simulink model "tx2"  (R2022a)
settings: Solver=FixedStepDiscrete  StartTime=0.0  StopTime=3.1e6  FixedStep=1  RelTol=1e-3
undefined symbols (not defined in the file or in its folder): rom_bf1, rom_bf2, rom_bf3, rom_bf4, rom_bf5, rom_bf6, rom_bf7, rom_bf8, rom_pilot_tt
libraries: hdlsllib x809, whdlutilities x460, whdlmod x104, whdledac x26, simulink x3
(part 2 of 27)

== system tx2/Subsystem1 ==
  process_data : Inport
  process_valid : Inport  Port=2
  BF : Subsystem
      settings: PortSchema="{\"entries\":[{\"content\":{\"sides\":[{\"content\":{\"connectorIds\":[\"In1\",\"In2\"]},\"type\":\"ConnectorPlacement.EquallySpacedRectSide\",\"uuid\":\"594cb7fb-008e-4551-8b9f-b11ed50deaba\"},{\"content\":{\"connectorIds\":[\"Out1\",\"Out2\",\"Out3\"],\"side\":\"RIGHT\"},\"type\":\"ConnectorPlacement.EquallySpacedRectSide\",\"uuid\":\"93ae86ad-1f5c-4115-9520-3a1a0cabfd8c\"},{\"content\":{\"connectorIds\":[\"In3\",\"In4\"],\"side\":\"TOP\"},\"type\":\"ConnectorPlacement.EquallySpacedRectSide\",\"uuid\":\"1fce8a66-8094-4bbb-b964-246637a8c1f4\"},{\"content\":{\"connectorIds\":[],\"side\":\"BOTTOM\"},\"type\":\"ConnectorPlacement.EquallySpacedRectSide\",\"uuid\":\"d45d1c11-e328-4038-90b1-bd9740dff9db\"}]},\"type\":\"ConnectorPlacement.EquallySpacedConnector\",\"uuid\":\"0bd8d214-ca11-4ecb-a7f0-3e13fd4fb1b3\"}],\"packageUris\":[\"http://schema.mathworks.com/mf0/Connector/R2020b\"],\"version\":\"1.0\"}"
  Bus Creator : BusCreator  Inputs=8
  Mux : Mux  Inputs=8
  OFDM_process1 : Subsystem  mask{cp=72}
      mask prompts: cp "the length of cp"
      mask DialogControl ParameterGroupVar Prompt: 参数
  bit_level : Subsystem
  mapping_process_L1 : Subsystem
      settings: PortSchema="{\"entries\":[{\"content\":{\"sides\":[{\"content\":{\"connectorIds\":[\"In1\",\"In2\"]},\"type\":\"ConnectorPlacement.EquallySpacedRectSide\",\"uuid\":\"660ebed9-a9a7-400e-a1e1-2a3bed22b258\"},{\"content\":{\"connectorIds\":[\"Out1\",\"Out2\"],\"side\":\"RIGHT\"},\"type\":\"ConnectorPlacement.EquallySpacedRectSide\",\"uuid\":\"141e197b-598d-477b-8a8c-cee3f2454319\"},{\"content\":{\"connectorIds\":[\"Out3\",\"Out4\"],\"side\":\"TOP\"},\"type\":\"ConnectorPlacement.EquallySpacedRectSide\",\"uuid\":\"c80a2ec3-9c02-4c14-8d74-14079e138b72\"}]},\"type\":\"ConnectorPlacement.EquallySpacedConnector\",\"uuid\":\"42120fb8-a7c5-4b68-b1ff-3dfc935ed9da\"}],\"packageUris\":[\"http://schema.mathworks.com/mf0/Connector/R2020b\"],\"version\":\"1.0\"}"
  OFDM_bf : Outport  PortDimensions=8
  OFDM_ctrl_bf : Outport  Port=2  OutDataTypeStr=Bus: BUSOFDM2
  wires:
  bit_level/2("bit_level_ctrl_process ") -> mapping_process_L1/2(mapping_ctrl)  "bit_level_ctrl"
  process_data/1 -> bit_level/1(process_data)
  mapping_process_L1/4(RB_id) -> BF/3(RB_id)  "RB_id_L1"
  mapping_process_L1/2(ctrl_mapping) -> BF/2(BF_data_ctrl)  "ctrl_mapping"
  mapping_process_L1/3(RB_ctrl) -> BF/4(RB_id_ctrl)  "RB_ctrl"
  bit_level/1(bit_level_process) -> mapping_process_L1/1(data_in)  "bit_level_process1"
  mapping_process_L1/1(data_out) -> BF/1(layer_data_in1)  "mapping_data_L1"
  process_valid/1 -> bit_level/2(process_valid)
  OFDM_process1/15(OFDM_bf8) -> Mux/8
  OFDM_process1/8(OFDM_ctrl_bf4) -> Bus Creator/4  "L4"
  OFDM_process1/1(OFDM_bf1) -> Mux/1
  OFDM_process1/5(OFDM_bf3) -> Mux/3
  Bus Creator/1 -> OFDM_ctrl_bf/1
  Mux/1 -> OFDM_bf/1
  BF/2(BF_ctrl) -> OFDM_process1/2(BF_ctrl)  "BF_ctrl"
  OFDM_process1/16(OFDM_ctrl_bf8) -> Bus Creator/8  "L8"
  OFDM_process1/10(OFDM_ctrl_bf5) -> Bus Creator/5  "L5"
  OFDM_process1/14(OFDM_ctrl_bf7) -> Bus Creator/7  "L7"
  OFDM_process1/12(OFDM_ctrl_bf6) -> Bus Creator/6  "L6"
  OFDM_process1/11(OFDM_bf6) -> Mux/6
  OFDM_process1/13(OFDM_bf7) -> Mux/7
  OFDM_process1/4(OFDM_ctrl_bf2) -> Bus Creator/2  "L2"
  OFDM_process1/3(OFDM_bf2) -> Mux/2
  OFDM_process1/7(OFDM_bf4) -> Mux/4
  OFDM_process1/9(OFDM_bf5) -> Mux/5
  OFDM_process1/2(OFDM_ctrl_bf1) -> Bus Creator/1  "L1"
  OFDM_process1/6(OFDM_ctrl_bf3) -> Bus Creator/3  "L3"
  BF/1(process_bf) -> OFDM_process1/1(process_bf)  "process_bf"

== system tx2/Subsystem10 ==
  process_data : Inport
  process_valid : Inport  Port=2
  BF : Subsystem
      settings: PortSchema="{\"entries\":[{\"content\":{\"sides\":[{\"content\":{\"connectorIds\":[\"In1\",\"In2\"]},\"type\":\"ConnectorPlacement.EquallySpacedRectSide\",\"uuid\":\"594cb7fb-008e-4551-8b9f-b11ed50deaba\"},{\"content\":{\"connectorIds\":[\"Out1\",\"Out2\",\"Out3\"],\"side\":\"RIGHT\"},\"type\":\"ConnectorPlacement.EquallySpacedRectSide\",\"uuid\":\"93ae86ad-1f5c-4115-9520-3a1a0cabfd8c\"},{\"content\":{\"connectorIds\":[\"In3\",\"In4\"],\"side\":\"TOP\"},\"type\":\"ConnectorPlacement.EquallySpacedRectSide\",\"uuid\":\"1fce8a66-8094-4bbb-b964-246637a8c1f4\"},{\"content\":{\"connectorIds\":[],\"side\":\"BOTTOM\"},\"type\":\"ConnectorPlacement.EquallySpacedRectSide\",\"uuid\":\"d45d1c11-e328-4038-90b1-bd9740dff9db\"}]},\"type\":\"ConnectorPlacement.EquallySpacedConnector\",\"uuid\":\"0bd8d214-ca11-4ecb-a7f0-3e13fd4fb1b3\"}],\"packageUris\":[\"http://schema.mathworks.com/mf0/Connector/R2020b\"],\"version\":\"1.0\"}"
  Bus Creator : BusCreator  Inputs=8
  Mux : Mux  Inputs=8
  OFDM_process1 : Subsystem  mask{cp=72}
      mask prompts: cp "the length of cp"
      mask DialogControl ParameterGroupVar Prompt: 参数
  bit_level : Subsystem
  mapping_process_L1 : Subsystem
      settings: PortSchema="{\"entries\":[{\"content\":{\"sides\":[{\"content\":{\"connectorIds\":[\"In1\",\"In2\"]},\"type\":\"ConnectorPlacement.EquallySpacedRectSide\",\"uuid\":\"660ebed9-a9a7-400e-a1e1-2a3bed22b258\"},{\"content\":{\"connectorIds\":[\"Out1\",\"Out2\"],\"side\":\"RIGHT\"},\"type\":\"ConnectorPlacement.EquallySpacedRectSide\",\"uuid\":\"141e197b-598d-477b-8a8c-cee3f2454319\"},{\"content\":{\"connectorIds\":[\"Out3\",\"Out4\"],\"side\":\"TOP\"},\"type\":\"ConnectorPlacement.EquallySpacedRectSide\",\"uuid\":\"c80a2ec3-9c02-4c14-8d74-14079e138b72\"}]},\"type\":\"ConnectorPlacement.EquallySpacedConnector\",\"uuid\":\"42120fb8-a7c5-4b68-b1ff-3dfc935ed9da\"}],\"packageUris\":[\"http://schema.mathworks.com/mf0/Connector/R2020b\"],\"version\":\"1.0\"}"
  OFDM_bf : Outport  PortDimensions=8
  OFDM_ctrl_bf : Outport  Port=2  OutDataTypeStr=Bus: BUSOFDM2
  wires:
  BF/1(process_bf) -> OFDM_process1/1(process_bf)  "process_bf"
  OFDM_process1/6(OFDM_ctrl_bf3) -> Bus Creator/3  "L3"
  OFDM_process1/2(OFDM_ctrl_bf1) -> Bus Creator/1  "L1"
  OFDM_process1/9(OFDM_bf5) -> Mux/5
  OFDM_process1/7(OFDM_bf4) -> Mux/4
  OFDM_process1/3(OFDM_bf2) -> Mux/2
  OFDM_process1/4(OFDM_ctrl_bf2) -> Bus Creator/2  "L2"
  OFDM_process1/13(OFDM_bf7) -> Mux/7
  OFDM_process1/11(OFDM_bf6) -> Mux/6
  OFDM_process1/12(OFDM_ctrl_bf6) -> Bus Creator/6  "L6"
  OFDM_process1/14(OFDM_ctrl_bf7) -> Bus Creator/7  "L7"
  OFDM_process1/10(OFDM_ctrl_bf5) -> Bus Creator/5  "L5"
  OFDM_process1/16(OFDM_ctrl_bf8) -> Bus Creator/8  "L8"
  BF/2(BF_ctrl) -> OFDM_process1/2(BF_ctrl)  "BF_ctrl"
  Mux/1 -> OFDM_bf/1
  Bus Creator/1 -> OFDM_ctrl_bf/1
  OFDM_process1/5(OFDM_bf3) -> Mux/3
  OFDM_process1/1(OFDM_bf1) -> Mux/1
  OFDM_process1/8(OFDM_ctrl_bf4) -> Bus Creator/4  "L4"
  OFDM_process1/15(OFDM_bf8) -> Mux/8
  process_valid/1 -> bit_level/2(process_valid)
  mapping_process_L1/1(data_out) -> BF/1(layer_data_in1)  "mapping_data_L1"
  bit_level/1(bit_level_process) -> mapping_process_L1/1(data_in)  "bit_level_process1"
  mapping_process_L1/3(RB_ctrl) -> BF/4(RB_id_ctrl)  "RB_ctrl"
  mapping_process_L1/2(ctrl_mapping) -> BF/2(BF_data_ctrl)  "ctrl_mapping"
  mapping_process_L1/4(RB_id) -> BF/3(RB_id)  "RB_id_L1"
  process_data/1 -> bit_level/1(process_data)
  bit_level/2("bit_level_ctrl_process ") -> mapping_process_L1/2(mapping_ctrl)  "bit_level_ctrl"

== system tx2/Subsystem11 ==
  process_data : Inport
  process_valid : Inport  Port=2
  BF : Subsystem
      settings: PortSchema="{\"entries\":[{\"content\":{\"sides\":[{\"content\":{\"connectorIds\":[\"In1\",\"In2\"]},\"type\":\"ConnectorPlacement.EquallySpacedRectSide\",\"uuid\":\"594cb7fb-008e-4551-8b9f-b11ed50deaba\"},{\"content\":{\"connectorIds\":[\"Out1\",\"Out2\",\"Out3\"],\"side\":\"RIGHT\"},\"type\":\"ConnectorPlacement.EquallySpacedRectSide\",\"uuid\":\"93ae86ad-1f5c-4115-9520-3a1a0cabfd8c\"},{\"content\":{\"connectorIds\":[\"In3\",\"In4\"],\"side\":\"TOP\"},\"type\":\"ConnectorPlacement.EquallySpacedRectSide\",\"uuid\":\"1fce8a66-8094-4bbb-b964-246637a8c1f4\"},{\"content\":{\"connectorIds\":[],\"side\":\"BOTTOM\"},\"type\":\"ConnectorPlacement.EquallySpacedRectSide\",\"uuid\":\"d45d1c11-e328-4038-90b1-bd9740dff9db\"}]},\"type\":\"ConnectorPlacement.EquallySpacedConnector\",\"uuid\":\"0bd8d214-ca11-4ecb-a7f0-3e13fd4fb1b3\"}],\"packageUris\":[\"http://schema.mathworks.com/mf0/Connector/R2020b\"],\"version\":\"1.0\"}"
  Bus Creator : BusCreator  Inputs=8
  Mux : Mux  Inputs=8
  OFDM_process1 : Subsystem  mask{cp=72}
      mask prompts: cp "the length of cp"
      mask DialogControl ParameterGroupVar Prompt: 参数
  bit_level : Subsystem
  mapping_process_L1 : Subsystem
      settings: PortSchema="{\"entries\":[{\"content\":{\"sides\":[{\"content\":{\"connectorIds\":[\"In1\",\"In2\"]},\"type\":\"ConnectorPlacement.EquallySpacedRectSide\",\"uuid\":\"660ebed9-a9a7-400e-a1e1-2a3bed22b258\"},{\"content\":{\"connectorIds\":[\"Out1\",\"Out2\"],\"side\":\"RIGHT\"},\"type\":\"ConnectorPlacement.EquallySpacedRectSide\",\"uuid\":\"141e197b-598d-477b-8a8c-cee3f2454319\"},{\"content\":{\"connectorIds\":[\"Out3\",\"Out4\"],\"side\":\"TOP\"},\"type\":\"ConnectorPlacement.EquallySpacedRectSide\",\"uuid\":\"c80a2ec3-9c02-4c14-8d74-14079e138b72\"}]},\"type\":\"ConnectorPlacement.EquallySpacedConnector\",\"uuid\":\"42120fb8-a7c5-4b68-b1ff-3dfc935ed9da\"}],\"packageUris\":[\"http://schema.mathworks.com/mf0/Connector/R2020b\"],\"version\":\"1.0\"}"
  OFDM_bf : Outport  PortDimensions=8
  OFDM_ctrl_bf : Outport  Port=2  OutDataTypeStr=Bus: BUSOFDM2
  wires:
  bit_level/2("bit_level_ctrl_process ") -> mapping_process_L1/2(mapping_ctrl)  "bit_level_ctrl"
  process_data/1 -> bit_level/1(process_data)
  mapping_process_L1/4(RB_id) -> BF/3(RB_id)  "RB_id_L1"
  mapping_process_L1/2(ctrl_mapping) -> BF/2(BF_data_ctrl)  "ctrl_mapping"
  mapping_process_L1/3(RB_ctrl) -> BF/4(RB_id_ctrl)  "RB_ctrl"
  bit_level/1(bit_level_process) -> mapping_process_L1/1(data_in)  "bit_level_process1"
  mapping_process_L1/1(data_out) -> BF/1(layer_data_in1)  "mapping_data_L1"
  process_valid/1 -> bit_level/2(process_valid)
  OFDM_process1/15(OFDM_bf8) -> Mux/8
  OFDM_process1/8(OFDM_ctrl_bf4) -> Bus Creator/4  "L4"
  OFDM_process1/1(OFDM_bf1) -> Mux/1
  OFDM_process1/5(OFDM_bf3) -> Mux/3
  Bus Creator/1 -> OFDM_ctrl_bf/1
  Mux/1 -> OFDM_bf/1
  BF/2(BF_ctrl) -> OFDM_process1/2(BF_ctrl)  "BF_ctrl"
  OFDM_process1/16(OFDM_ctrl_bf8) -> Bus Creator/8  "L8"
  OFDM_process1/10(OFDM_ctrl_bf5) -> Bus Creator/5  "L5"
  OFDM_process1/14(OFDM_ctrl_bf7) -> Bus Creator/7  "L7"
  OFDM_process1/12(OFDM_ctrl_bf6) -> Bus Creator/6  "L6"
  OFDM_process1/11(OFDM_bf6) -> Mux/6
  OFDM_process1/13(OFDM_bf7) -> Mux/7
  OFDM_process1/4(OFDM_ctrl_bf2) -> Bus Creator/2  "L2"
  OFDM_process1/3(OFDM_bf2) -> Mux/2
  OFDM_process1/7(OFDM_bf4) -> Mux/4
  OFDM_process1/9(OFDM_bf5) -> Mux/5
  OFDM_process1/2(OFDM_ctrl_bf1) -> Bus Creator/1  "L1"
  OFDM_process1/6(OFDM_ctrl_bf3) -> Bus Creator/3  "L3"
  BF/1(process_bf) -> OFDM_process1/1(process_bf)  "process_bf"

== system tx2/Subsystem12 ==
  process_data : Inport
  process_valid : Inport  Port=2
  BF : Subsystem
      settings: PortSchema="{\"entries\":[{\"content\":{\"sides\":[{\"content\":{\"connectorIds\":[\"In1\",\"In2\"]},\"type\":\"ConnectorPlacement.EquallySpacedRectSide\",\"uuid\":\"594cb7fb-008e-4551-8b9f-b11ed50deaba\"},{\"content\":{\"connectorIds\":[\"Out1\",\"Out2\",\"Out3\"],\"side\":\"RIGHT\"},\"type\":\"ConnectorPlacement.EquallySpacedRectSide\",\"uuid\":\"93ae86ad-1f5c-4115-9520-3a1a0cabfd8c\"},{\"content\":{\"connectorIds\":[\"In3\",\"In4\"],\"side\":\"TOP\"},\"type\":\"ConnectorPlacement.EquallySpacedRectSide\",\"uuid\":\"1fce8a66-8094-4bbb-b964-246637a8c1f4\"},{\"content\":{\"connectorIds\":[],\"side\":\"BOTTOM\"},\"type\":\"ConnectorPlacement.EquallySpacedRectSide\",\"uuid\":\"d45d1c11-e328-4038-90b1-bd9740dff9db\"}]},\"type\":\"ConnectorPlacement.EquallySpacedConnector\",\"uuid\":\"0bd8d214-ca11-4ecb-a7f0-3e13fd4fb1b3\"}],\"packageUris\":[\"http://schema.mathworks.com/mf0/Connector/R2020b\"],\"version\":\"1.0\"}"
  Bus Creator : BusCreator  Inputs=8
  Mux : Mux  Inputs=8
  OFDM_process1 : Subsystem  mask{cp=72}
      mask prompts: cp "the length of cp"
      mask DialogControl ParameterGroupVar Prompt: 参数
  bit_level : Subsystem
  mapping_process_L1 : Subsystem
      settings: PortSchema="{\"entries\":[{\"content\":{\"sides\":[{\"content\":{\"connectorIds\":[\"In1\",\"In2\"]},\"type\":\"ConnectorPlacement.EquallySpacedRectSide\",\"uuid\":\"660ebed9-a9a7-400e-a1e1-2a3bed22b258\"},{\"content\":{\"connectorIds\":[\"Out1\",\"Out2\"],\"side\":\"RIGHT\"},\"type\":\"ConnectorPlacement.EquallySpacedRectSide\",\"uuid\":\"141e197b-598d-477b-8a8c-cee3f2454319\"},{\"content\":{\"connectorIds\":[\"Out3\",\"Out4\"],\"side\":\"TOP\"},\"type\":\"ConnectorPlacement.EquallySpacedRectSide\",\"uuid\":\"c80a2ec3-9c02-4c14-8d74-14079e138b72\"}]},\"type\":\"ConnectorPlacement.EquallySpacedConnector\",\"uuid\":\"42120fb8-a7c5-4b68-b1ff-3dfc935ed9da\"}],\"packageUris\":[\"http://schema.mathworks.com/mf0/Connector/R2020b\"],\"version\":\"1.0\"}"
  OFDM_bf : Outport  PortDimensions=8
  OFDM_ctrl_bf : Outport  Port=2  OutDataTypeStr=Bus: BUSOFDM2
  wires:
  BF/1(process_bf) -> OFDM_process1/1(process_bf)  "process_bf"
  OFDM_process1/6(OFDM_ctrl_bf3) -> Bus Creator/3  "L3"
  OFDM_process1/2(OFDM_ctrl_bf1) -> Bus Creator/1  "L1"
  OFDM_process1/9(OFDM_bf5) -> Mux/5
  OFDM_process1/7(OFDM_bf4) -> Mux/4
  OFDM_process1/3(OFDM_bf2) -> Mux/2
  OFDM_process1/4(OFDM_ctrl_bf2) -> Bus Creator/2  "L2"
  OFDM_process1/13(OFDM_bf7) -> Mux/7
  OFDM_process1/11(OFDM_bf6) -> Mux/6
  OFDM_process1/12(OFDM_ctrl_bf6) -> Bus Creator/6  "L6"
  OFDM_process1/14(OFDM_ctrl_bf7) -> Bus Creator/7  "L7"
  OFDM_process1/10(OFDM_ctrl_bf5) -> Bus Creator/5  "L5"
  OFDM_process1/16(OFDM_ctrl_bf8) -> Bus Creator/8  "L8"
  BF/2(BF_ctrl) -> OFDM_process1/2(BF_ctrl)  "BF_ctrl"
  Mux/1 -> OFDM_bf/1
  Bus Creator/1 -> OFDM_ctrl_bf/1
  OFDM_process1/5(OFDM_bf3) -> Mux/3
  OFDM_process1/1(OFDM_bf1) -> Mux/1
  OFDM_process1/8(OFDM_ctrl_bf4) -> Bus Creator/4  "L4"
  OFDM_process1/15(OFDM_bf8) -> Mux/8
  process_valid/1 -> bit_level/2(process_valid)
  mapping_process_L1/1(data_out) -> BF/1(layer_data_in1)  "mapping_data_L1"
  bit_level/1(bit_level_process) -> mapping_process_L1/1(data_in)  "bit_level_process1"
  mapping_process_L1/3(RB_ctrl) -> BF/4(RB_id_ctrl)  "RB_ctrl"
  mapping_process_L1/2(ctrl_mapping) -> BF/2(BF_data_ctrl)  "ctrl_mapping"
  mapping_process_L1/4(RB_id) -> BF/3(RB_id)  "RB_id_L1"
  process_data/1 -> bit_level/1(process_data)
  bit_level/2("bit_level_ctrl_process ") -> mapping_process_L1/2(mapping_ctrl)  "bit_level_ctrl"

== system tx2/Subsystem13 ==
  process_data : Inport
  process_valid : Inport  Port=2
  BF : Subsystem
      settings: PortSchema="{\"entries\":[{\"content\":{\"sides\":[{\"content\":{\"connectorIds\":[\"In1\",\"In2\"]},\"type\":\"ConnectorPlacement.EquallySpacedRectSide\",\"uuid\":\"594cb7fb-008e-4551-8b9f-b11ed50deaba\"},{\"content\":{\"connectorIds\":[\"Out1\",\"Out2\",\"Out3\"],\"side\":\"RIGHT\"},\"type\":\"ConnectorPlacement.EquallySpacedRectSide\",\"uuid\":\"93ae86ad-1f5c-4115-9520-3a1a0cabfd8c\"},{\"content\":{\"connectorIds\":[\"In3\",\"In4\"],\"side\":\"TOP\"},\"type\":\"ConnectorPlacement.EquallySpacedRectSide\",\"uuid\":\"1fce8a66-8094-4bbb-b964-246637a8c1f4\"},{\"content\":{\"connectorIds\":[],\"side\":\"BOTTOM\"},\"type\":\"ConnectorPlacement.EquallySpacedRectSide\",\"uuid\":\"d45d1c11-e328-4038-90b1-bd9740dff9db\"}]},\"type\":\"ConnectorPlacement.EquallySpacedConnector\",\"uuid\":\"0bd8d214-ca11-4ecb-a7f0-3e13fd4fb1b3\"}],\"packageUris\":[\"http://schema.mathworks.com/mf0/Connector/R2020b\"],\"version\":\"1.0\"}"
  Bus Creator : BusCreator  Inputs=8
  Mux : Mux  Inputs=8
  OFDM_process1 : Subsystem  mask{cp=72}
      mask prompts: cp "the length of cp"
      mask DialogControl ParameterGroupVar Prompt: 参数
  bit_level : Subsystem
  mapping_process_L1 : Subsystem
      settings: PortSchema="{\"entries\":[{\"content\":{\"sides\":[{\"content\":{\"connectorIds\":[\"In1\",\"In2\"]},\"type\":\"ConnectorPlacement.EquallySpacedRectSide\",\"uuid\":\"660ebed9-a9a7-400e-a1e1-2a3bed22b258\"},{\"content\":{\"connectorIds\":[\"Out1\",\"Out2\"],\"side\":\"RIGHT\"},\"type\":\"ConnectorPlacement.EquallySpacedRectSide\",\"uuid\":\"141e197b-598d-477b-8a8c-cee3f2454319\"},{\"content\":{\"connectorIds\":[\"Out3\",\"Out4\"],\"side\":\"TOP\"},\"type\":\"ConnectorPlacement.EquallySpacedRectSide\",\"uuid\":\"c80a2ec3-9c02-4c14-8d74-14079e138b72\"}]},\"type\":\"ConnectorPlacement.EquallySpacedConnector\",\"uuid\":\"42120fb8-a7c5-4b68-b1ff-3dfc935ed9da\"}],\"packageUris\":[\"http://schema.mathworks.com/mf0/Connector/R2020b\"],\"version\":\"1.0\"}"
  OFDM_bf : Outport  PortDimensions=8
  OFDM_ctrl_bf : Outport  Port=2  OutDataTypeStr=Bus: BUSOFDM2
  wires:
  bit_level/2("bit_level_ctrl_process ") -> mapping_process_L1/2(mapping_ctrl)  "bit_level_ctrl"
  process_data/1 -> bit_level/1(process_data)
  mapping_process_L1/4(RB_id) -> BF/3(RB_id)  "RB_id_L1"
  mapping_process_L1/2(ctrl_mapping) -> BF/2(BF_data_ctrl)  "ctrl_mapping"
  mapping_process_L1/3(RB_ctrl) -> BF/4(RB_id_ctrl)  "RB_ctrl"
  bit_level/1(bit_level_process) -> mapping_process_L1/1(data_in)  "bit_level_process1"
  mapping_process_L1/1(data_out) -> BF/1(layer_data_in1)  "mapping_data_L1"
  process_valid/1 -> bit_level/2(process_valid)
  OFDM_process1/15(OFDM_bf8) -> Mux/8
  OFDM_process1/8(OFDM_ctrl_bf4) -> Bus Creator/4  "L4"
  OFDM_process1/1(OFDM_bf1) -> Mux/1
  OFDM_process1/5(OFDM_bf3) -> Mux/3
  Bus Creator/1 -> OFDM_ctrl_bf/1
  Mux/1 -> OFDM_bf/1
  BF/2(BF_ctrl) -> OFDM_process1/2(BF_ctrl)  "BF_ctrl"
  OFDM_process1/16(OFDM_ctrl_bf8) -> Bus Creator/8  "L8"
  OFDM_process1/10(OFDM_ctrl_bf5) -> Bus Creator/5  "L5"
  OFDM_process1/14(OFDM_ctrl_bf7) -> Bus Creator/7  "L7"
  OFDM_process1/12(OFDM_ctrl_bf6) -> Bus Creator/6  "L6"
  OFDM_process1/11(OFDM_bf6) -> Mux/6
  OFDM_process1/13(OFDM_bf7) -> Mux/7
  OFDM_process1/4(OFDM_ctrl_bf2) -> Bus Creator/2  "L2"
  OFDM_process1/3(OFDM_bf2) -> Mux/2
  OFDM_process1/7(OFDM_bf4) -> Mux/4
  OFDM_process1/9(OFDM_bf5) -> Mux/5
  OFDM_process1/2(OFDM_ctrl_bf1) -> Bus Creator/1  "L1"
  OFDM_process1/6(OFDM_ctrl_bf3) -> Bus Creator/3  "L3"
  BF/1(process_bf) -> OFDM_process1/1(process_bf)  "process_bf"

== system tx2/Subsystem2 ==
  process_data : Inport
  process_valid : Inport  Port=2
  BF : Subsystem
      settings: PortSchema="{\"entries\":[{\"content\":{\"sides\":[{\"content\":{\"connectorIds\":[\"In1\",\"In2\"]},\"type\":\"ConnectorPlacement.EquallySpacedRectSide\",\"uuid\":\"594cb7fb-008e-4551-8b9f-b11ed50deaba\"},{\"content\":{\"connectorIds\":[\"Out1\",\"Out2\",\"Out3\"],\"side\":\"RIGHT\"},\"type\":\"ConnectorPlacement.EquallySpacedRectSide\",\"uuid\":\"93ae86ad-1f5c-4115-9520-3a1a0cabfd8c\"},{\"content\":{\"connectorIds\":[\"In3\",\"In4\"],\"side\":\"TOP\"},\"type\":\"ConnectorPlacement.EquallySpacedRectSide\",\"uuid\":\"1fce8a66-8094-4bbb-b964-246637a8c1f4\"},{\"content\":{\"connectorIds\":[],\"side\":\"BOTTOM\"},\"type\":\"ConnectorPlacement.EquallySpacedRectSide\",\"uuid\":\"d45d1c11-e328-4038-90b1-bd9740dff9db\"}]},\"type\":\"ConnectorPlacement.EquallySpacedConnector\",\"uuid\":\"0bd8d214-ca11-4ecb-a7f0-3e13fd4fb1b3\"}],\"packageUris\":[\"http://schema.mathworks.com/mf0/Connector/R2020b\"],\"version\":\"1.0\"}"
  Bus Creator : BusCreator  Inputs=8
  Mux : Mux  Inputs=8
  OFDM_process1 : Subsystem  mask{cp=72}
      mask prompts: cp "the length of cp"
      mask DialogControl ParameterGroupVar Prompt: 参数
  bit_level : Subsystem
  mapping_process_L1 : Subsystem
      settings: PortSchema="{\"entries\":[{\"content\":{\"sides\":[{\"content\":{\"connectorIds\":[\"In1\",\"In2\"]},\"type\":\"ConnectorPlacement.EquallySpacedRectSide\",\"uuid\":\"660ebed9-a9a7-400e-a1e1-2a3bed22b258\"},{\"content\":{\"connectorIds\":[\"Out1\",\"Out2\"],\"side\":\"RIGHT\"},\"type\":\"ConnectorPlacement.EquallySpacedRectSide\",\"uuid\":\"141e197b-598d-477b-8a8c-cee3f2454319\"},{\"content\":{\"connectorIds\":[\"Out3\",\"Out4\"],\"side\":\"TOP\"},\"type\":\"ConnectorPlacement.EquallySpacedRectSide\",\"uuid\":\"c80a2ec3-9c02-4c14-8d74-14079e138b72\"}]},\"type\":\"ConnectorPlacement.EquallySpacedConnector\",\"uuid\":\"42120fb8-a7c5-4b68-b1ff-3dfc935ed9da\"}],\"packageUris\":[\"http://schema.mathworks.com/mf0/Connector/R2020b\"],\"version\":\"1.0\"}"
  OFDM_bf : Outport  PortDimensions=8
  OFDM_ctrl_bf : Outport  Port=2  OutDataTypeStr=Bus: BUSOFDM2
  wires:
  BF/1(process_bf) -> OFDM_process1/1(process_bf)  "process_bf"
  OFDM_process1/6(OFDM_ctrl_bf3) -> Bus Creator/3  "L3"
  OFDM_process1/2(OFDM_ctrl_bf1) -> Bus Creator/1  "L1"
  OFDM_process1/9(OFDM_bf5) -> Mux/5
  OFDM_process1/7(OFDM_bf4) -> Mux/4
  OFDM_process1/3(OFDM_bf2) -> Mux/2
  OFDM_process1/4(OFDM_ctrl_bf2) -> Bus Creator/2  "L2"
  OFDM_process1/13(OFDM_bf7) -> Mux/7
  OFDM_process1/11(OFDM_bf6) -> Mux/6
  OFDM_process1/12(OFDM_ctrl_bf6) -> Bus Creator/6  "L6"
  OFDM_process1/14(OFDM_ctrl_bf7) -> Bus Creator/7  "L7"
  OFDM_process1/10(OFDM_ctrl_bf5) -> Bus Creator/5  "L5"
  OFDM_process1/16(OFDM_ctrl_bf8) -> Bus Creator/8  "L8"
  BF/2(BF_ctrl) -> OFDM_process1/2(BF_ctrl)  "BF_ctrl"
  Mux/1 -> OFDM_bf/1
  Bus Creator/1 -> OFDM_ctrl_bf/1
  OFDM_process1/5(OFDM_bf3) -> Mux/3
  OFDM_process1/1(OFDM_bf1) -> Mux/1
  OFDM_process1/8(OFDM_ctrl_bf4) -> Bus Creator/4  "L4"
  OFDM_process1/15(OFDM_bf8) -> Mux/8
  process_valid/1 -> bit_level/2(process_valid)
  mapping_process_L1/1(data_out) -> BF/1(layer_data_in1)  "mapping_data_L1"
  bit_level/1(bit_level_process) -> mapping_process_L1/1(data_in)  "bit_level_process1"
  mapping_process_L1/3(RB_ctrl) -> BF/4(RB_id_ctrl)  "RB_ctrl"
  mapping_process_L1/2(ctrl_mapping) -> BF/2(BF_data_ctrl)  "ctrl_mapping"
  mapping_process_L1/4(RB_id) -> BF/3(RB_id)  "RB_id_L1"
  process_data/1 -> bit_level/1(process_data)
  bit_level/2("bit_level_ctrl_process ") -> mapping_process_L1/2(mapping_ctrl)  "bit_level_ctrl"

== system tx2/Subsystem3 ==
  process_data : Inport
  process_valid : Inport  Port=2
  BF : Subsystem
      settings: PortSchema="{\"entries\":[{\"content\":{\"sides\":[{\"content\":{\"connectorIds\":[\"In1\",\"In2\"]},\"type\":\"ConnectorPlacement.EquallySpacedRectSide\",\"uuid\":\"594cb7fb-008e-4551-8b9f-b11ed50deaba\"},{\"content\":{\"connectorIds\":[\"Out1\",\"Out2\",\"Out3\"],\"side\":\"RIGHT\"},\"type\":\"ConnectorPlacement.EquallySpacedRectSide\",\"uuid\":\"93ae86ad-1f5c-4115-9520-3a1a0cabfd8c\"},{\"content\":{\"connectorIds\":[\"In3\",\"In4\"],\"side\":\"TOP\"},\"type\":\"ConnectorPlacement.EquallySpacedRectSide\",\"uuid\":\"1fce8a66-8094-4bbb-b964-246637a8c1f4\"},{\"content\":{\"connectorIds\":[],\"side\":\"BOTTOM\"},\"type\":\"ConnectorPlacement.EquallySpacedRectSide\",\"uuid\":\"d45d1c11-e328-4038-90b1-bd9740dff9db\"}]},\"type\":\"ConnectorPlacement.EquallySpacedConnector\",\"uuid\":\"0bd8d214-ca11-4ecb-a7f0-3e13fd4fb1b3\"}],\"packageUris\":[\"http://schema.mathworks.com/mf0/Connector/R2020b\"],\"version\":\"1.0\"}"
  Bus Creator : BusCreator  Inputs=8
  Mux : Mux  Inputs=8
  OFDM_process1 : Subsystem  mask{cp=72}
      mask prompts: cp "the length of cp"
      mask DialogControl ParameterGroupVar Prompt: 参数
  bit_level : Subsystem
  mapping_process_L1 : Subsystem
      settings: PortSchema="{\"entries\":[{\"content\":{\"sides\":[{\"content\":{\"connectorIds\":[\"In1\",\"In2\"]},\"type\":\"ConnectorPlacement.EquallySpacedRectSide\",\"uuid\":\"660ebed9-a9a7-400e-a1e1-2a3bed22b258\"},{\"content\":{\"connectorIds\":[\"Out1\",\"Out2\"],\"side\":\"RIGHT\"},\"type\":\"ConnectorPlacement.EquallySpacedRectSide\",\"uuid\":\"141e197b-598d-477b-8a8c-cee3f2454319\"},{\"content\":{\"connectorIds\":[\"Out3\",\"Out4\"],\"side\":\"TOP\"},\"type\":\"ConnectorPlacement.EquallySpacedRectSide\",\"uuid\":\"c80a2ec3-9c02-4c14-8d74-14079e138b72\"}]},\"type\":\"ConnectorPlacement.EquallySpacedConnector\",\"uuid\":\"42120fb8-a7c5-4b68-b1ff-3dfc935ed9da\"}],\"packageUris\":[\"http://schema.mathworks.com/mf0/Connector/R2020b\"],\"version\":\"1.0\"}"
  OFDM_bf : Outport  PortDimensions=8
  OFDM_ctrl_bf : Outport  Port=2  OutDataTypeStr=Bus: BUSOFDM2
  wires:
  bit_level/2("bit_level_ctrl_process ") -> mapping_process_L1/2(mapping_ctrl)  "bit_level_ctrl"
  process_data/1 -> bit_level/1(process_data)
  mapping_process_L1/4(RB_id) -> BF/3(RB_id)  "RB_id_L1"
  mapping_process_L1/2(ctrl_mapping) -> BF/2(BF_data_ctrl)  "ctrl_mapping"
  mapping_process_L1/3(RB_ctrl) -> BF/4(RB_id_ctrl)  "RB_ctrl"
  bit_level/1(bit_level_process) -> mapping_process_L1/1(data_in)  "bit_level_process1"
  mapping_process_L1/1(data_out) -> BF/1(layer_data_in1)  "mapping_data_L1"
  process_valid/1 -> bit_level/2(process_valid)
  OFDM_process1/15(OFDM_bf8) -> Mux/8
  OFDM_process1/8(OFDM_ctrl_bf4) -> Bus Creator/4  "L4"
  OFDM_process1/1(OFDM_bf1) -> Mux/1
  OFDM_process1/5(OFDM_bf3) -> Mux/3
  Bus Creator/1 -> OFDM_ctrl_bf/1
  Mux/1 -> OFDM_bf/1
  BF/2(BF_ctrl) -> OFDM_process1/2(BF_ctrl)  "BF_ctrl"
  OFDM_process1/16(OFDM_ctrl_bf8) -> Bus Creator/8  "L8"
  OFDM_process1/10(OFDM_ctrl_bf5) -> Bus Creator/5  "L5"
  OFDM_process1/14(OFDM_ctrl_bf7) -> Bus Creator/7  "L7"
  OFDM_process1/12(OFDM_ctrl_bf6) -> Bus Creator/6  "L6"
  OFDM_process1/11(OFDM_bf6) -> Mux/6
  OFDM_process1/13(OFDM_bf7) -> Mux/7
  OFDM_process1/4(OFDM_ctrl_bf2) -> Bus Creator/2  "L2"
  OFDM_process1/3(OFDM_bf2) -> Mux/2
  OFDM_process1/7(OFDM_bf4) -> Mux/4
  OFDM_process1/9(OFDM_bf5) -> Mux/5
  OFDM_process1/2(OFDM_ctrl_bf1) -> Bus Creator/1  "L1"
  OFDM_process1/6(OFDM_ctrl_bf3) -> Bus Creator/3  "L3"
  BF/1(process_bf) -> OFDM_process1/1(process_bf)  "process_bf"

== system tx2/Subsystem4 ==
  process_data : Inport
  process_valid : Inport  Port=2
  BF : Subsystem
      settings: PortSchema="{\"entries\":[{\"content\":{\"sides\":[{\"content\":{\"connectorIds\":[\"In1\",\"In2\"]},\"type\":\"ConnectorPlacement.EquallySpacedRectSide\",\"uuid\":\"594cb7fb-008e-4551-8b9f-b11ed50deaba\"},{\"content\":{\"connectorIds\":[\"Out1\",\"Out2\",\"Out3\"],\"side\":\"RIGHT\"},\"type\":\"ConnectorPlacement.EquallySpacedRectSide\",\"uuid\":\"93ae86ad-1f5c-4115-9520-3a1a0cabfd8c\"},{\"content\":{\"connectorIds\":[\"In3\",\"In4\"],\"side\":\"TOP\"},\"type\":\"ConnectorPlacement.EquallySpacedRectSide\",\"uuid\":\"1fce8a66-8094-4bbb-b964-246637a8c1f4\"},{\"content\":{\"connectorIds\":[],\"side\":\"BOTTOM\"},\"type\":\"ConnectorPlacement.EquallySpacedRectSide\",\"uuid\":\"d45d1c11-e328-4038-90b1-bd9740dff9db\"}]},\"type\":\"ConnectorPlacement.EquallySpacedConnector\",\"uuid\":\"0bd8d214-ca11-4ecb-a7f0-3e13fd4fb1b3\"}],\"packageUris\":[\"http://schema.mathworks.com/mf0/Connector/R2020b\"],\"version\":\"1.0\"}"
  Bus Creator : BusCreator  Inputs=8
  Mux : Mux  Inputs=8
  OFDM_process1 : Subsystem  mask{cp=72}
      mask prompts: cp "the length of cp"
      mask DialogControl ParameterGroupVar Prompt: 参数
  bit_level : Subsystem
  mapping_process_L1 : Subsystem
      settings: PortSchema="{\"entries\":[{\"content\":{\"sides\":[{\"content\":{\"connectorIds\":[\"In1\",\"In2\"]},\"type\":\"ConnectorPlacement.EquallySpacedRectSide\",\"uuid\":\"660ebed9-a9a7-400e-a1e1-2a3bed22b258\"},{\"content\":{\"connectorIds\":[\"Out1\",\"Out2\"],\"side\":\"RIGHT\"},\"type\":\"ConnectorPlacement.EquallySpacedRectSide\",\"uuid\":\"141e197b-598d-477b-8a8c-cee3f2454319\"},{\"content\":{\"connectorIds\":[\"Out3\",\"Out4\"],\"side\":\"TOP\"},\"type\":\"ConnectorPlacement.EquallySpacedRectSide\",\"uuid\":\"c80a2ec3-9c02-4c14-8d74-14079e138b72\"}]},\"type\":\"ConnectorPlacement.EquallySpacedConnector\",\"uuid\":\"42120fb8-a7c5-4b68-b1ff-3dfc935ed9da\"}],\"packageUris\":[\"http://schema.mathworks.com/mf0/Connector/R2020b\"],\"version\":\"1.0\"}"
  OFDM_bf : Outport  PortDimensions=8
  OFDM_ctrl_bf : Outport  Port=2  OutDataTypeStr=Bus: BUSOFDM2
  wires:
  BF/1(process_bf) -> OFDM_process1/1(process_bf)  "process_bf"
  OFDM_process1/6(OFDM_ctrl_bf3) -> Bus Creator/3  "L3"
  OFDM_process1/2(OFDM_ctrl_bf1) -> Bus Creator/1  "L1"
  OFDM_process1/9(OFDM_bf5) -> Mux/5
  OFDM_process1/7(OFDM_bf4) -> Mux/4
  OFDM_process1/3(OFDM_bf2) -> Mux/2
  OFDM_process1/4(OFDM_ctrl_bf2) -> Bus Creator/2  "L2"
  OFDM_process1/13(OFDM_bf7) -> Mux/7
  OFDM_process1/11(OFDM_bf6) -> Mux/6
  OFDM_process1/12(OFDM_ctrl_bf6) -> Bus Creator/6  "L6"
  OFDM_process1/14(OFDM_ctrl_bf7) -> Bus Creator/7  "L7"
  OFDM_process1/10(OFDM_ctrl_bf5) -> Bus Creator/5  "L5"
  OFDM_process1/16(OFDM_ctrl_bf8) -> Bus Creator/8  "L8"
  BF/2(BF_ctrl) -> OFDM_process1/2(BF_ctrl)  "BF_ctrl"
  Mux/1 -> OFDM_bf/1
  Bus Creator/1 -> OFDM_ctrl_bf/1
  OFDM_process1/5(OFDM_bf3) -> Mux/3
  OFDM_process1/1(OFDM_bf1) -> Mux/1
  OFDM_process1/8(OFDM_ctrl_bf4) -> Bus Creator/4  "L4"
  OFDM_process1/15(OFDM_bf8) -> Mux/8
  process_valid/1 -> bit_level/2(process_valid)
  mapping_process_L1/1(data_out) -> BF/1(layer_data_in1)  "mapping_data_L1"
  bit_level/1(bit_level_process) -> mapping_process_L1/1(data_in)  "bit_level_process1"
  mapping_process_L1/3(RB_ctrl) -> BF/4(RB_id_ctrl)  "RB_ctrl"
  mapping_process_L1/2(ctrl_mapping) -> BF/2(BF_data_ctrl)  "ctrl_mapping"
  mapping_process_L1/4(RB_id) -> BF/3(RB_id)  "RB_id_L1"
  process_data/1 -> bit_level/1(process_data)
  bit_level/2("bit_level_ctrl_process ") -> mapping_process_L1/2(mapping_ctrl)  "bit_level_ctrl"

== system tx2/Subsystem5 ==
  process_data : Inport
  process_valid : Inport  Port=2
  BF : Subsystem
      settings: PortSchema="{\"entries\":[{\"content\":{\"sides\":[{\"content\":{\"connectorIds\":[\"In1\",\"In2\"]},\"type\":\"ConnectorPlacement.EquallySpacedRectSide\",\"uuid\":\"594cb7fb-008e-4551-8b9f-b11ed50deaba\"},{\"content\":{\"connectorIds\":[\"Out1\",\"Out2\",\"Out3\"],\"side\":\"RIGHT\"},\"type\":\"ConnectorPlacement.EquallySpacedRectSide\",\"uuid\":\"93ae86ad-1f5c-4115-9520-3a1a0cabfd8c\"},{\"content\":{\"connectorIds\":[\"In3\",\"In4\"],\"side\":\"TOP\"},\"type\":\"ConnectorPlacement.EquallySpacedRectSide\",\"uuid\":\"1fce8a66-8094-4bbb-b964-246637a8c1f4\"},{\"content\":{\"connectorIds\":[],\"side\":\"BOTTOM\"},\"type\":\"ConnectorPlacement.EquallySpacedRectSide\",\"uuid\":\"d45d1c11-e328-4038-90b1-bd9740dff9db\"}]},\"type\":\"ConnectorPlacement.EquallySpacedConnector\",\"uuid\":\"0bd8d214-ca11-4ecb-a7f0-3e13fd4fb1b3\"}],\"packageUris\":[\"http://schema.mathworks.com/mf0/Connector/R2020b\"],\"version\":\"1.0\"}"
  Bus Creator : BusCreator  Inputs=8
  Mux : Mux  Inputs=8
  OFDM_process1 : Subsystem  mask{cp=72}
      mask prompts: cp "the length of cp"
      mask DialogControl ParameterGroupVar Prompt: 参数
  bit_level : Subsystem
  mapping_process_L1 : Subsystem
      settings: PortSchema="{\"entries\":[{\"content\":{\"sides\":[{\"content\":{\"connectorIds\":[\"In1\",\"In2\"]},\"type\":\"ConnectorPlacement.EquallySpacedRectSide\",\"uuid\":\"660ebed9-a9a7-400e-a1e1-2a3bed22b258\"},{\"content\":{\"connectorIds\":[\"Out1\",\"Out2\"],\"side\":\"RIGHT\"},\"type\":\"ConnectorPlacement.EquallySpacedRectSide\",\"uuid\":\"141e197b-598d-477b-8a8c-cee3f2454319\"},{\"content\":{\"connectorIds\":[\"Out3\",\"Out4\"],\"side\":\"TOP\"},\"type\":\"ConnectorPlacement.EquallySpacedRectSide\",\"uuid\":\"c80a2ec3-9c02-4c14-8d74-14079e138b72\"}]},\"type\":\"ConnectorPlacement.EquallySpacedConnector\",\"uuid\":\"42120fb8-a7c5-4b68-b1ff-3dfc935ed9da\"}],\"packageUris\":[\"http://schema.mathworks.com/mf0/Connector/R2020b\"],\"version\":\"1.0\"}"
  OFDM_bf : Outport  PortDimensions=8
  OFDM_ctrl_bf : Outport  Port=2  OutDataTypeStr=Bus: BUSOFDM2
  wires:
  bit_level/2("bit_level_ctrl_process ") -> mapping_process_L1/2(mapping_ctrl)  "bit_level_ctrl"
  process_data/1 -> bit_level/1(process_data)
  mapping_process_L1/4(RB_id) -> BF/3(RB_id)  "RB_id_L1"
  mapping_process_L1/2(ctrl_mapping) -> BF/2(BF_data_ctrl)  "ctrl_mapping"
  mapping_process_L1/3(RB_ctrl) -> BF/4(RB_id_ctrl)  "RB_ctrl"
  bit_level/1(bit_level_process) -> mapping_process_L1/1(data_in)  "bit_level_process1"
  mapping_process_L1/1(data_out) -> BF/1(layer_data_in1)  "mapping_data_L1"
  process_valid/1 -> bit_level/2(process_valid)
  OFDM_process1/15(OFDM_bf8) -> Mux/8
  OFDM_process1/8(OFDM_ctrl_bf4) -> Bus Creator/4  "L4"
  OFDM_process1/1(OFDM_bf1) -> Mux/1
  OFDM_process1/5(OFDM_bf3) -> Mux/3
  Bus Creator/1 -> OFDM_ctrl_bf/1
  Mux/1 -> OFDM_bf/1
  BF/2(BF_ctrl) -> OFDM_process1/2(BF_ctrl)  "BF_ctrl"
  OFDM_process1/16(OFDM_ctrl_bf8) -> Bus Creator/8  "L8"
  OFDM_process1/10(OFDM_ctrl_bf5) -> Bus Creator/5  "L5"
  OFDM_process1/14(OFDM_ctrl_bf7) -> Bus Creator/7  "L7"
  OFDM_process1/12(OFDM_ctrl_bf6) -> Bus Creator/6  "L6"
  OFDM_process1/11(OFDM_bf6) -> Mux/6
  OFDM_process1/13(OFDM_bf7) -> Mux/7
  OFDM_process1/4(OFDM_ctrl_bf2) -> Bus Creator/2  "L2"
  OFDM_process1/3(OFDM_bf2) -> Mux/2
  OFDM_process1/7(OFDM_bf4) -> Mux/4
  OFDM_process1/9(OFDM_bf5) -> Mux/5
  OFDM_process1/2(OFDM_ctrl_bf1) -> Bus Creator/1  "L1"
  OFDM_process1/6(OFDM_ctrl_bf3) -> Bus Creator/3  "L3"
  BF/1(process_bf) -> OFDM_process1/1(process_bf)  "process_bf"

== system tx2/Subsystem6 ==
  process_data : Inport
  process_valid : Inport  Port=2
  BF : Subsystem
      settings: PortSchema="{\"entries\":[{\"content\":{\"sides\":[{\"content\":{\"connectorIds\":[\"In1\",\"In2\"]},\"type\":\"ConnectorPlacement.EquallySpacedRectSide\",\"uuid\":\"594cb7fb-008e-4551-8b9f-b11ed50deaba\"},{\"content\":{\"connectorIds\":[\"Out1\",\"Out2\",\"Out3\"],\"side\":\"RIGHT\"},\"type\":\"ConnectorPlacement.EquallySpacedRectSide\",\"uuid\":\"93ae86ad-1f5c-4115-9520-3a1a0cabfd8c\"},{\"content\":{\"connectorIds\":[\"In3\",\"In4\"],\"side\":\"TOP\"},\"type\":\"ConnectorPlacement.EquallySpacedRectSide\",\"uuid\":\"1fce8a66-8094-4bbb-b964-246637a8c1f4\"},{\"content\":{\"connectorIds\":[],\"side\":\"BOTTOM\"},\"type\":\"ConnectorPlacement.EquallySpacedRectSide\",\"uuid\":\"d45d1c11-e328-4038-90b1-bd9740dff9db\"}]},\"type\":\"ConnectorPlacement.EquallySpacedConnector\",\"uuid\":\"0bd8d214-ca11-4ecb-a7f0-3e13fd4fb1b3\"}],\"packageUris\":[\"http://schema.mathworks.com/mf0/Connector/R2020b\"],\"version\":\"1.0\"}"
  Bus Creator : BusCreator  Inputs=8
  Mux : Mux  Inputs=8
  OFDM_process1 : Subsystem  mask{cp=72}
      mask prompts: cp "the length of cp"
      mask DialogControl ParameterGroupVar Prompt: 参数
  bit_level : Subsystem
  mapping_process_L1 : Subsystem
      settings: PortSchema="{\"entries\":[{\"content\":{\"sides\":[{\"content\":{\"connectorIds\":[\"In1\",\"In2\"]},\"type\":\"ConnectorPlacement.EquallySpacedRectSide\",\"uuid\":\"660ebed9-a9a7-400e-a1e1-2a3bed22b258\"},{\"content\":{\"connectorIds\":[\"Out1\",\"Out2\"],\"side\":\"RIGHT\"},\"type\":\"ConnectorPlacement.EquallySpacedRectSide\",\"uuid\":\"141e197b-598d-477b-8a8c-cee3f2454319\"},{\"content\":{\"connectorIds\":[\"Out3\",\"Out4\"],\"side\":\"TOP\"},\"type\":\"ConnectorPlacement.EquallySpacedRectSide\",\"uuid\":\"c80a2ec3-9c02-4c14-8d74-14079e138b72\"}]},\"type\":\"ConnectorPlacement.EquallySpacedConnector\",\"uuid\":\"42120fb8-a7c5-4b68-b1ff-3dfc935ed9da\"}],\"packageUris\":[\"http://schema.mathworks.com/mf0/Connector/R2020b\"],\"version\":\"1.0\"}"
  OFDM_bf : Outport  PortDimensions=8
  OFDM_ctrl_bf : Outport  Port=2  OutDataTypeStr=Bus: BUSOFDM2
  wires:
  BF/1(process_bf) -> OFDM_process1/1(process_bf)  "process_bf"
  OFDM_process1/6(OFDM_ctrl_bf3) -> Bus Creator/3  "L3"
  OFDM_process1/2(OFDM_ctrl_bf1) -> Bus Creator/1  "L1"
  OFDM_process1/9(OFDM_bf5) -> Mux/5
  OFDM_process1/7(OFDM_bf4) -> Mux/4
  OFDM_process1/3(OFDM_bf2) -> Mux/2
  OFDM_process1/4(OFDM_ctrl_bf2) -> Bus Creator/2  "L2"
  OFDM_process1/13(OFDM_bf7) -> Mux/7
  OFDM_process1/11(OFDM_bf6) -> Mux/6
  OFDM_process1/12(OFDM_ctrl_bf6) -> Bus Creator/6  "L6"
  OFDM_process1/14(OFDM_ctrl_bf7) -> Bus Creator/7  "L7"
  OFDM_process1/10(OFDM_ctrl_bf5) -> Bus Creator/5  "L5"
  OFDM_process1/16(OFDM_ctrl_bf8) -> Bus Creator/8  "L8"
  BF/2(BF_ctrl) -> OFDM_process1/2(BF_ctrl)  "BF_ctrl"
  Mux/1 -> OFDM_bf/1
  Bus Creator/1 -> OFDM_ctrl_bf/1
  OFDM_process1/5(OFDM_bf3) -> Mux/3
  OFDM_process1/1(OFDM_bf1) -> Mux/1
  OFDM_process1/8(OFDM_ctrl_bf4) -> Bus Creator/4  "L4"
  OFDM_process1/15(OFDM_bf8) -> Mux/8
  process_valid/1 -> bit_level/2(process_valid)
  mapping_process_L1/1(data_out) -> BF/1(layer_data_in1)  "mapping_data_L1"
  bit_level/1(bit_level_process) -> mapping_process_L1/1(data_in)  "bit_level_process1"
  mapping_process_L1/3(RB_ctrl) -> BF/4(RB_id_ctrl)  "RB_ctrl"
  mapping_process_L1/2(ctrl_mapping) -> BF/2(BF_data_ctrl)  "ctrl_mapping"
  mapping_process_L1/4(RB_id) -> BF/3(RB_id)  "RB_id_L1"
  process_data/1 -> bit_level/1(process_data)
  bit_level/2("bit_level_ctrl_process ") -> mapping_process_L1/2(mapping_ctrl)  "bit_level_ctrl"

== system tx2/Subsystem7 ==
  process_data : Inport
  process_valid : Inport  Port=2
  BF : Subsystem
      settings: PortSchema="{\"entries\":[{\"content\":{\"sides\":[{\"content\":{\"connectorIds\":[\"In1\",\"In2\"]},\"type\":\"ConnectorPlacement.EquallySpacedRectSide\",\"uuid\":\"594cb7fb-008e-4551-8b9f-b11ed50deaba\"},{\"content\":{\"connectorIds\":[\"Out1\",\"Out2\",\"Out3\"],\"side\":\"RIGHT\"},\"type\":\"ConnectorPlacement.EquallySpacedRectSide\",\"uuid\":\"93ae86ad-1f5c-4115-9520-3a1a0cabfd8c\"},{\"content\":{\"connectorIds\":[\"In3\",\"In4\"],\"side\":\"TOP\"},\"type\":\"ConnectorPlacement.EquallySpacedRectSide\",\"uuid\":\"1fce8a66-8094-4bbb-b964-246637a8c1f4\"},{\"content\":{\"connectorIds\":[],\"side\":\"BOTTOM\"},\"type\":\"ConnectorPlacement.EquallySpacedRectSide\",\"uuid\":\"d45d1c11-e328-4038-90b1-bd9740dff9db\"}]},\"type\":\"ConnectorPlacement.EquallySpacedConnector\",\"uuid\":\"0bd8d214-ca11-4ecb-a7f0-3e13fd4fb1b3\"}],\"packageUris\":[\"http://schema.mathworks.com/mf0/Connector/R2020b\"],\"version\":\"1.0\"}"
  Bus Creator : BusCreator  Inputs=8
  Mux : Mux  Inputs=8
  OFDM_process1 : Subsystem  mask{cp=72}
      mask prompts: cp "the length of cp"
      mask DialogControl ParameterGroupVar Prompt: 参数
  bit_level : Subsystem
  mapping_process_L1 : Subsystem
      settings: PortSchema="{\"entries\":[{\"content\":{\"sides\":[{\"content\":{\"connectorIds\":[\"In1\",\"In2\"]},\"type\":\"ConnectorPlacement.EquallySpacedRectSide\",\"uuid\":\"660ebed9-a9a7-400e-a1e1-2a3bed22b258\"},{\"content\":{\"connectorIds\":[\"Out1\",\"Out2\"],\"side\":\"RIGHT\"},\"type\":\"ConnectorPlacement.EquallySpacedRectSide\",\"uuid\":\"141e197b-598d-477b-8a8c-cee3f2454319\"},{\"content\":{\"connectorIds\":[\"Out3\",\"Out4\"],\"side\":\"TOP\"},\"type\":\"ConnectorPlacement.EquallySpacedRectSide\",\"uuid\":\"c80a2ec3-9c02-4c14-8d74-14079e138b72\"}]},\"type\":\"ConnectorPlacement.EquallySpacedConnector\",\"uuid\":\"42120fb8-a7c5-4b68-b1ff-3dfc935ed9da\"}],\"packageUris\":[\"http://schema.mathworks.com/mf0/Connector/R2020b\"],\"version\":\"1.0\"}"
  OFDM_bf : Outport  PortDimensions=8
  OFDM_ctrl_bf : Outport  Port=2  OutDataTypeStr=Bus: BUSOFDM2
  wires:
  bit_level/2("bit_level_ctrl_process ") -> mapping_process_L1/2(mapping_ctrl)  "bit_level_ctrl"
  process_data/1 -> bit_level/1(process_data)
  mapping_process_L1/4(RB_id) -> BF/3(RB_id)  "RB_id_L1"
  mapping_process_L1/2(ctrl_mapping) -> BF/2(BF_data_ctrl)  "ctrl_mapping"
  mapping_process_L1/3(RB_ctrl) -> BF/4(RB_id_ctrl)  "RB_ctrl"
  bit_level/1(bit_level_process) -> mapping_process_L1/1(data_in)  "bit_level_process1"
  mapping_process_L1/1(data_out) -> BF/1(layer_data_in1)  "mapping_data_L1"
  process_valid/1 -> bit_level/2(process_valid)
  OFDM_process1/15(OFDM_bf8) -> Mux/8
  OFDM_process1/8(OFDM_ctrl_bf4) -> Bus Creator/4  "L4"
  OFDM_process1/1(OFDM_bf1) -> Mux/1
  OFDM_process1/5(OFDM_bf3) -> Mux/3
  Bus Creator/1 -> OFDM_ctrl_bf/1
  Mux/1 -> OFDM_bf/1
  BF/2(BF_ctrl) -> OFDM_process1/2(BF_ctrl)  "BF_ctrl"
  OFDM_process1/16(OFDM_ctrl_bf8) -> Bus Creator/8  "L8"
  OFDM_process1/10(OFDM_ctrl_bf5) -> Bus Creator/5  "L5"
  OFDM_process1/14(OFDM_ctrl_bf7) -> Bus Creator/7  "L7"
  OFDM_process1/12(OFDM_ctrl_bf6) -> Bus Creator/6  "L6"
  OFDM_process1/11(OFDM_bf6) -> Mux/6
  OFDM_process1/13(OFDM_bf7) -> Mux/7
  OFDM_process1/4(OFDM_ctrl_bf2) -> Bus Creator/2  "L2"
  OFDM_process1/3(OFDM_bf2) -> Mux/2
  OFDM_process1/7(OFDM_bf4) -> Mux/4
  OFDM_process1/9(OFDM_bf5) -> Mux/5
  OFDM_process1/2(OFDM_ctrl_bf1) -> Bus Creator/1  "L1"
  OFDM_process1/6(OFDM_ctrl_bf3) -> Bus Creator/3  "L3"
  BF/1(process_bf) -> OFDM_process1/1(process_bf)  "process_bf"

== system tx2/Subsystem8 ==
  process_data : Inport
  process_valid : Inport  Port=2
  BF : Subsystem
      settings: PortSchema="{\"entries\":[{\"content\":{\"sides\":[{\"content\":{\"connectorIds\":[\"In1\",\"In2\"]},\"type\":\"ConnectorPlacement.EquallySpacedRectSide\",\"uuid\":\"594cb7fb-008e-4551-8b9f-b11ed50deaba\"},{\"content\":{\"connectorIds\":[\"Out1\",\"Out2\",\"Out3\"],\"side\":\"RIGHT\"},\"type\":\"ConnectorPlacement.EquallySpacedRectSide\",\"uuid\":\"93ae86ad-1f5c-4115-9520-3a1a0cabfd8c\"},{\"content\":{\"connectorIds\":[\"In3\",\"In4\"],\"side\":\"TOP\"},\"type\":\"ConnectorPlacement.EquallySpacedRectSide\",\"uuid\":\"1fce8a66-8094-4bbb-b964-246637a8c1f4\"},{\"content\":{\"connectorIds\":[],\"side\":\"BOTTOM\"},\"type\":\"ConnectorPlacement.EquallySpacedRectSide\",\"uuid\":\"d45d1c11-e328-4038-90b1-bd9740dff9db\"}]},\"type\":\"ConnectorPlacement.EquallySpacedConnector\",\"uuid\":\"0bd8d214-ca11-4ecb-a7f0-3e13fd4fb1b3\"}],\"packageUris\":[\"http://schema.mathworks.com/mf0/Connector/R2020b\"],\"version\":\"1.0\"}"
  Bus Creator : BusCreator  Inputs=8
  Mux : Mux  Inputs=8
  OFDM_process1 : Subsystem  mask{cp=72}
      mask prompts: cp "the length of cp"
      mask DialogControl ParameterGroupVar Prompt: 参数
  bit_level : Subsystem
  mapping_process_L1 : Subsystem
      settings: PortSchema="{\"entries\":[{\"content\":{\"sides\":[{\"content\":{\"connectorIds\":[\"In1\",\"In2\"]},\"type\":\"ConnectorPlacement.EquallySpacedRectSide\",\"uuid\":\"660ebed9-a9a7-400e-a1e1-2a3bed22b258\"},{\"content\":{\"connectorIds\":[\"Out1\",\"Out2\"],\"side\":\"RIGHT\"},\"type\":\"ConnectorPlacement.EquallySpacedRectSide\",\"uuid\":\"141e197b-598d-477b-8a8c-cee3f2454319\"},{\"content\":{\"connectorIds\":[\"Out3\",\"Out4\"],\"side\":\"TOP\"},\"type\":\"ConnectorPlacement.EquallySpacedRectSide\",\"uuid\":\"c80a2ec3-9c02-4c14-8d74-14079e138b72\"}]},\"type\":\"ConnectorPlacement.EquallySpacedConnector\",\"uuid\":\"42120fb8-a7c5-4b68-b1ff-3dfc935ed9da\"}],\"packageUris\":[\"http://schema.mathworks.com/mf0/Connector/R2020b\"],\"version\":\"1.0\"}"
  OFDM_bf : Outport  PortDimensions=8
  OFDM_ctrl_bf : Outport  Port=2  OutDataTypeStr=Bus: BUSOFDM2
  wires:
  BF/1(process_bf) -> OFDM_process1/1(process_bf)  "process_bf"
  OFDM_process1/6(OFDM_ctrl_bf3) -> Bus Creator/3  "L3"
  OFDM_process1/2(OFDM_ctrl_bf1) -> Bus Creator/1  "L1"
  OFDM_process1/9(OFDM_bf5) -> Mux/5
  OFDM_process1/7(OFDM_bf4) -> Mux/4
  OFDM_process1/3(OFDM_bf2) -> Mux/2
  OFDM_process1/4(OFDM_ctrl_bf2) -> Bus Creator/2  "L2"
  OFDM_process1/13(OFDM_bf7) -> Mux/7
  OFDM_process1/11(OFDM_bf6) -> Mux/6
  OFDM_process1/12(OFDM_ctrl_bf6) -> Bus Creator/6  "L6"
  OFDM_process1/14(OFDM_ctrl_bf7) -> Bus Creator/7  "L7"
  OFDM_process1/10(OFDM_ctrl_bf5) -> Bus Creator/5  "L5"
  OFDM_process1/16(OFDM_ctrl_bf8) -> Bus Creator/8  "L8"
  BF/2(BF_ctrl) -> OFDM_process1/2(BF_ctrl)  "BF_ctrl"
  Mux/1 -> OFDM_bf/1
  Bus Creator/1 -> OFDM_ctrl_bf/1
  OFDM_process1/5(OFDM_bf3) -> Mux/3
  OFDM_process1/1(OFDM_bf1) -> Mux/1
  OFDM_process1/8(OFDM_ctrl_bf4) -> Bus Creator/4  "L4"
  OFDM_process1/15(OFDM_bf8) -> Mux/8
  process_valid/1 -> bit_level/2(process_valid)
  mapping_process_L1/1(data_out) -> BF/1(layer_data_in1)  "mapping_data_L1"
  bit_level/1(bit_level_process) -> mapping_process_L1/1(data_in)  "bit_level_process1"
  mapping_process_L1/3(RB_ctrl) -> BF/4(RB_id_ctrl)  "RB_ctrl"
  mapping_process_L1/2(ctrl_mapping) -> BF/2(BF_data_ctrl)  "ctrl_mapping"
  mapping_process_L1/4(RB_id) -> BF/3(RB_id)  "RB_id_L1"
  process_data/1 -> bit_level/1(process_data)
  bit_level/2("bit_level_ctrl_process ") -> mapping_process_L1/2(mapping_ctrl)  "bit_level_ctrl"

== system tx2/Subsystem9 ==
  process_data : Inport
  process_valid : Inport  Port=2
  BF : Subsystem
      settings: PortSchema="{\"entries\":[{\"content\":{\"sides\":[{\"content\":{\"connectorIds\":[\"In1\",\"In2\"]},\"type\":\"ConnectorPlacement.EquallySpacedRectSide\",\"uuid\":\"594cb7fb-008e-4551-8b9f-b11ed50deaba\"},{\"content\":{\"connectorIds\":[\"Out1\",\"Out2\",\"Out3\"],\"side\":\"RIGHT\"},\"type\":\"ConnectorPlacement.EquallySpacedRectSide\",\"uuid\":\"93ae86ad-1f5c-4115-9520-3a1a0cabfd8c\"},{\"content\":{\"connectorIds\":[\"In3\",\"In4\"],\"side\":\"TOP\"},\"type\":\"ConnectorPlacement.EquallySpacedRectSide\",\"uuid\":\"1fce8a66-8094-4bbb-b964-246637a8c1f4\"},{\"content\":{\"connectorIds\":[],\"side\":\"BOTTOM\"},\"type\":\"ConnectorPlacement.EquallySpacedRectSide\",\"uuid\":\"d45d1c11-e328-4038-90b1-bd9740dff9db\"}]},\"type\":\"ConnectorPlacement.EquallySpacedConnector\",\"uuid\":\"0bd8d214-ca11-4ecb-a7f0-3e13fd4fb1b3\"}],\"packageUris\":[\"http://schema.mathworks.com/mf0/Connector/R2020b\"],\"version\":\"1.0\"}"
  Bus Creator : BusCreator  Inputs=8
  Mux : Mux  Inputs=8
  OFDM_process1 : Subsystem  mask{cp=72}
      mask prompts: cp "the length of cp"
      mask DialogControl ParameterGroupVar Prompt: 参数
  bit_level : Subsystem
  mapping_process_L1 : Subsystem
      settings: PortSchema="{\"entries\":[{\"content\":{\"sides\":[{\"content\":{\"connectorIds\":[\"In1\",\"In2\"]},\"type\":\"ConnectorPlacement.EquallySpacedRectSide\",\"uuid\":\"660ebed9-a9a7-400e-a1e1-2a3bed22b258\"},{\"content\":{\"connectorIds\":[\"Out1\",\"Out2\"],\"side\":\"RIGHT\"},\"type\":\"ConnectorPlacement.EquallySpacedRectSide\",\"uuid\":\"141e197b-598d-477b-8a8c-cee3f2454319\"},{\"content\":{\"connectorIds\":[\"Out3\",\"Out4\"],\"side\":\"TOP\"},\"type\":\"ConnectorPlacement.EquallySpacedRectSide\",\"uuid\":\"c80a2ec3-9c02-4c14-8d74-14079e138b72\"}]},\"type\":\"ConnectorPlacement.EquallySpacedConnector\",\"uuid\":\"42120fb8-a7c5-4b68-b1ff-3dfc935ed9da\"}],\"packageUris\":[\"http://schema.mathworks.com/mf0/Connector/R2020b\"],\"version\":\"1.0\"}"
  OFDM_bf : Outport  PortDimensions=8
  OFDM_ctrl_bf : Outport  Port=2  OutDataTypeStr=Bus: BUSOFDM2
  wires:
  bit_level/2("bit_level_ctrl_process ") -> mapping_process_L1/2(mapping_ctrl)  "bit_level_ctrl"
  process_data/1 -> bit_level/1(process_data)
  mapping_process_L1/4(RB_id) -> BF/3(RB_id)  "RB_id_L1"
  mapping_process_L1/2(ctrl_mapping) -> BF/2(BF_data_ctrl)  "ctrl_mapping"
  mapping_process_L1/3(RB_ctrl) -> BF/4(RB_id_ctrl)  "RB_ctrl"
  bit_level/1(bit_level_process) -> mapping_process_L1/1(data_in)  "bit_level_process1"
  mapping_process_L1/1(data_out) -> BF/1(layer_data_in1)  "mapping_data_L1"
  process_valid/1 -> bit_level/2(process_valid)
  OFDM_process1/15(OFDM_bf8) -> Mux/8
  OFDM_process1/8(OFDM_ctrl_bf4) -> Bus Creator/4  "L4"
  OFDM_process1/1(OFDM_bf1) -> Mux/1
  OFDM_process1/5(OFDM_bf3) -> Mux/3
  Bus Creator/1 -> OFDM_ctrl_bf/1
  Mux/1 -> OFDM_bf/1
  BF/2(BF_ctrl) -> OFDM_process1/2(BF_ctrl)  "BF_ctrl"
  OFDM_process1/16(OFDM_ctrl_bf8) -> Bus Creator/8  "L8"
  OFDM_process1/10(OFDM_ctrl_bf5) -> Bus Creator/5  "L5"
  OFDM_process1/14(OFDM_ctrl_bf7) -> Bus Creator/7  "L7"
  OFDM_process1/12(OFDM_ctrl_bf6) -> Bus Creator/6  "L6"
  OFDM_process1/11(OFDM_bf6) -> Mux/6
  OFDM_process1/13(OFDM_bf7) -> Mux/7
  OFDM_process1/4(OFDM_ctrl_bf2) -> Bus Creator/2  "L2"
  OFDM_process1/3(OFDM_bf2) -> Mux/2
  OFDM_process1/7(OFDM_bf4) -> Mux/4
  OFDM_process1/9(OFDM_bf5) -> Mux/5
  OFDM_process1/2(OFDM_ctrl_bf1) -> Bus Creator/1  "L1"
  OFDM_process1/6(OFDM_ctrl_bf3) -> Bus Creator/3  "L3"
  BF/1(process_bf) -> OFDM_process1/1(process_bf)  "process_bf"
